simulink model "negative_input"  (R2025b)
settings: Solver=ode5  StartTime=0.0  StopTime=45  FixedStep=0.001  RelTol=1e-3
undefined symbols (not defined in the file): degs2rpm, kd, ki, kp, National_Instruments, PCI, rdp, rpm2degs, sens, simul, step_gain, tl, Ts
libraries: sldrtlib x3, simulink x3
settings Model: SimulationMode=external  ExtModeTrigDuration=45001  Creator=fasoloandr  LastModifiedBy=Enrico
settings DataIOCC: ReturnWorkspaceOutputs=off
settings HardwareCC: ProdBitPerLong=64.0  ProdHWDeviceType=Intel->x86-64 (Linux 64)
settings RTWCC: SystemTargetFile=sldrt.tlc  TemplateMakefile=sldrt.tmf  RTWCompilerOptimization=on  Description=Simulink Desktop Real-Time
settings CodeAppCC: MaxIdLength=95.0
settings SimulinkDesktopRealTimeCC: ExtModeTransport=0.0  ExtModeStaticAllocSize=1000000.0  TargetLibSuffix=_sldrt.a  TargetPreCompLibLocation=D:\Programmi (D)\MATLAB\R2025b\toolbox\sldrt\lib\win64  MultiwordLength=2048.0  DynamicStringBufferSize=256.0  ParMdlRefBuildCompliant=on  PreserveMATLABNamespacesInGeneratedCode=on  SubcomponentCodeInterfacePackaging=Reusable function

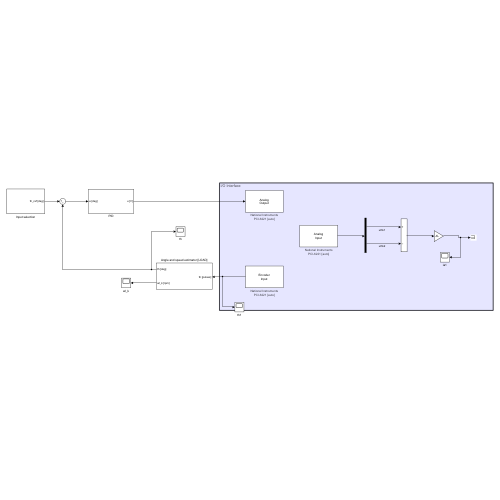
[thumbnail: Simulink's stored preview of the top-level diagram]
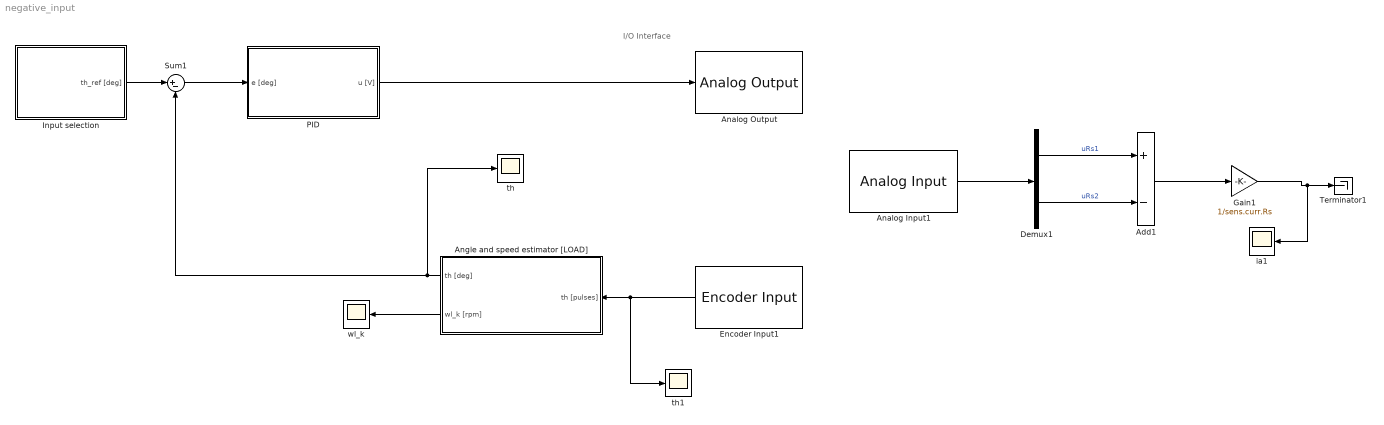
== system negative_input ==
  note: I/O Interface
  Add1 : Sum  Inputs=+-
  Analog Input1 : sldrtlib/Analog Input  SampleTime=-1  MaxMissedTicks=10  ShowMissedTicks=off  YieldWhenWaiting=off  DrvName=National_Instruments/PCI-6221  DrvAddress=4294967295  DrvOptions=[0 0 0 2 0]  Channels=[1,2]  RangeMode=1  VoltRange=1  DataType=1
      settings: AttributesFormatString=National Instruments\nPCI-6221 [auto]
  Analog Output : sldrtlib/Analog Output  SampleTime=-1  MaxMissedTicks=10  ShowMissedTicks=off  YieldWhenWaiting=off  DrvName=National_Instruments/PCI-6221  DrvAddress=4294967295  DrvOptions=[0 0 0 2 0]  Channels=1  RangeMode=1  VoltRange=1  InitialValue=[0]  FinalValue=[0]
      settings: AttributesFormatString=National Instruments\nPCI-6221 [auto]
  Angle and speed estimator [LOAD] : Subsystem
  Demux1 : Demux  Outputs=2
  Encoder Input1 : sldrtlib/Encoder Input  SampleTime=-1  MaxMissedTicks=10  ShowMissedTicks=off  YieldWhenWaiting=off  DrvName=National_Instruments/PCI-6221  DrvAddress=4294967295  DrvOptions=[0 0 0 2 0]  Channels=1  QuadMode=3  IndexPulse=1  InputFilter=Inf  DataType=1
      settings: AttributesFormatString=National Instruments\nPCI-6221 [auto]
  Gain1 : Gain  Gain=1/sens.curr.Rs
  Input selection : Subsystem
  PID : Subsystem
  Sum1 : Sum  Inputs=|+-
  Terminator1 : Terminator
  ia1 : Scope
      settings: ActiveDisplayYMinimum=-0.03865  ActiveDisplayYMaximum=0.30896  DataLoggingVariableName=ScopeData2
  th : Scope
      settings: ActiveDisplayYMinimum=-8437.4775  ActiveDisplayYMaximum=75937.2975
  th1 : Scope
      settings: ActiveDisplayYMinimum=-46874.875  ActiveDisplayYMaximum=421873.875
  wl_k : Scope
      settings: ActiveDisplayYMinimum=-56.64383  ActiveDisplayYMaximum=509.79443
  wires:
  Angle and speed estimator [LOAD]/1(th [deg]) -> th/1, Sum1/2
  Sum1/1 -> PID/1(e [deg])
  PID/1(u [V]) -> Analog Output/1
  Add1/1 -> Gain1/1
  Demux1/1 -> Add1/1  "uRs1"
  Demux1/2 -> Add1/2  "uRs2"
  Gain1/1 -> ia1/1, Terminator1/1
  Analog Input1/1 -> Demux1/1
  Encoder Input1/1 -> th1/1, Angle and speed estimator [LOAD]/1(th [pulses])
  Angle and speed estimator [LOAD]/2(wl_k [rpm]) -> wl_k/1
  Input selection/1(th_ref [deg]) -> Sum1/1

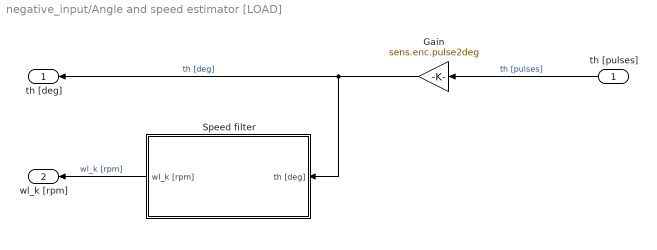
== system negative_input/Angle and speed estimator [LOAD] ==
  th [pulses] : Inport
  Gain : Gain  Gain=sens.enc.pulse2deg
  Speed filter : Subsystem
  th [deg] : Outport
  wl_k [rpm] : Outport  Port=2
  wires:
  Speed filter/1(wl_k [rpm]) -> wl_k [rpm]/1  "wl_k [rpm]"
  th [pulses]/1 -> Gain/1  "th [pulses]"
  Gain/1 -> Speed filter/1(th [deg]), th [deg]/1  "th [deg]"

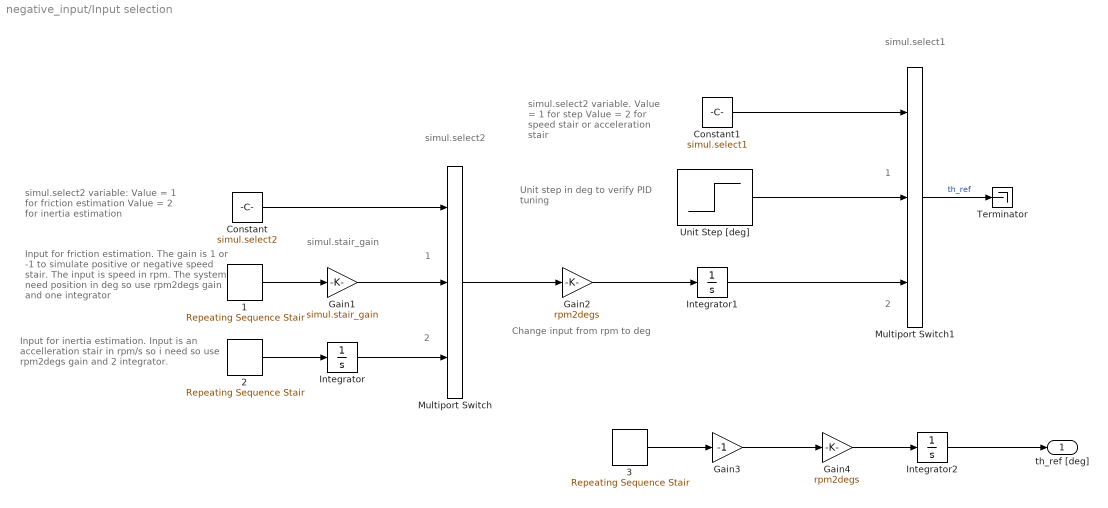
== system negative_input/Input selection ==
  note: Change input from rpm to deg
  note: Input for friction estimation. The gain
      | is 1 or -1 to simulate positive or negative
      | speed stair. The input is speed in rpm.
      | The system need position in deg so use
      | rpm2degs gain and one integrator
  note: Input for inertia estimation. Input is an
      | accelleration stair in rpm/s so i need so use
      | rpm2degs gain and 2 integrator.
  note: simul.select2 variable:
      | Value = 1 for friction estimation
      | Value = 2 for inertia estimation
  note: Unit step in deg to verify PID
      | tuning
  note: simul.select2 variable.
      | Value = 1 for step
      | Value = 2 for speed stair
      | or acceleration stair
  note: simul.select2
  note: simul.select1
  note: simul.stair_gain
  note: 1
  note: 2
  note: 1
  note: 2
  1 : simulink/Sources/Repeating Sequence Stair  OutValues=[50 100 150 200 250 300 350 400 450 450].'  tsamp=5  OutMin=[]  OutMax=[]  OutDataTypeStr=double  OutputDataTypeScalingMode=double  OutDataType=fixdt(0,8)  ConRadixGroup=Best Precision: Vector-wise  OutScaling=2^-12
  2 : simulink/Sources/Repeating Sequence Stair  OutValues=[450 -450].'  tsamp=1  OutMin=[]  OutMax=[]  OutDataTypeStr=double  OutputDataTypeScalingMode=double  OutDataType=fixdt(0,8)  ConRadixGroup=Best Precision: Vector-wise  OutScaling=2^-12
  3 : simulink/Sources/Repeating Sequence Stair  OutValues=[50 100 150 200 250 300 350 400 450 450].'  tsamp=5  OutMin=[]  OutMax=[]  OutDataTypeStr=double  OutputDataTypeScalingMode=double  OutDataType=fixdt(0,8)  ConRadixGroup=Best Precision: Vector-wise  OutScaling=2^-12
  Constant : Constant  Value=simul.select2
  Constant1 : Constant  Value=simul.select1
  Gain1 : Gain  Gain=simul.stair_gain
  Gain2 : Gain  Gain=rpm2degs
  Gain3 : Gain  Gain=-1
  Gain4 : Gain  Gain=rpm2degs
  Integrator : Integrator
  Integrator1 : Integrator
  Integrator2 : Integrator
  Multiport Switch : MultiPortSwitch  Inputs=2  SaturateOnIntegerOverflow=off  InputSameDT=off
  Multiport Switch1 : MultiPortSwitch  Inputs=2  SaturateOnIntegerOverflow=off  InputSameDT=off
  Terminator : Terminator
  Unit Step [deg] : Step  After=step_gain  SampleTime=Ts
  th_ref [deg] : Outport
  wires:
  Integrator1/1 -> Multiport Switch1/3
  Constant/1 -> Multiport Switch/1
  Gain1/1 -> Multiport Switch/2
  1/1 -> Gain1/1
  Gain2/1 -> Integrator1/1
  2/1 -> Integrator/1
  Unit Step [deg]/1 -> Multiport Switch1/2
  Constant1/1 -> Multiport Switch1/1
  Multiport Switch/1 -> Gain2/1
  Integrator/1 -> Multiport Switch/3
  3/1 -> Gain3/1
  Gain3/1 -> Gain4/1
  Gain4/1 -> Integrator2/1
  Integrator2/1 -> th_ref [deg]/1
  Multiport Switch1/1 -> Terminator/1  "th_ref"

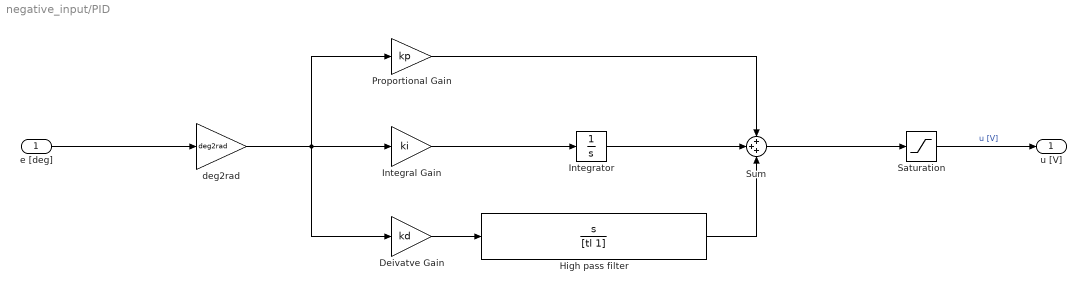
== system negative_input/PID ==
  e [deg] : Inport
  Deivatve Gain : Gain  Gain=kd
  High pass filter : TransferFcn  Numerator=[1 0]  Denominator=[tl 1]
  Integral Gain : Gain  Gain=ki
  Integrator : Integrator
  Proportional Gain : Gain  Gain=kp
  "Saturation " : Saturate  UpperLimit=10  LowerLimit=-10
  Sum : Sum  Inputs=+++
  deg2rad : Gain  Gain=deg2rad
  u [V] : Outport
  wires:
  Deivatve Gain/1 -> High pass filter/1
  e [deg]/1 -> deg2rad/1
  Integrator/1 -> Sum/2
  "Saturation "/1 -> u [V]/1  "u [V]"
  deg2rad/1 -> Deivatve Gain/1, Proportional Gain/1, Integral Gain/1
  High pass filter/1 -> Sum/3
  Integral Gain/1 -> Integrator/1
  Proportional Gain/1 -> Sum/1
  Sum/1 -> "Saturation "/1

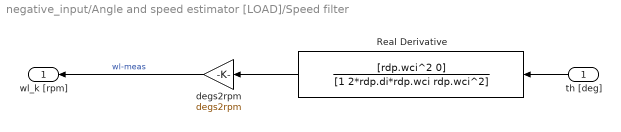
== system negative_input/Angle and speed estimator [LOAD]/Speed filter ==
  th [deg] : Inport
  Real Derivative : TransferFcn  Numerator=[rdp.wci^2 0]  Denominator=[1 2*rdp.di*rdp.wci rdp.wci^2]
  degs2rpm : Gain  Gain=degs2rpm
  wl_k [rpm] : Outport
  wires:
  th [deg]/1 -> Real Derivative/1
  degs2rpm/1 -> wl_k [rpm]/1  "wl-meas"
  Real Derivative/1 -> degs2rpm/1
